simulink model "fuck"  (R2016a)
settings: Solver=ode5  StartTime=0.0  StopTime=10  FixedStep=0.001  RelTol=1e-3
values from neighbouring files (symbols this model uses):
  LK1 = -LK1    [car.m]    (also in car_m.m = [-1 0;0 -1]')
  x0 = [1 3 2 1 3 2 4 5]'    [car.m]    (also in car_m.m = [0 0]')
  xd = [10 10]    [car_m.m]
libraries: simulink x3
settings Model: Creator=108  LastModifiedBy=108

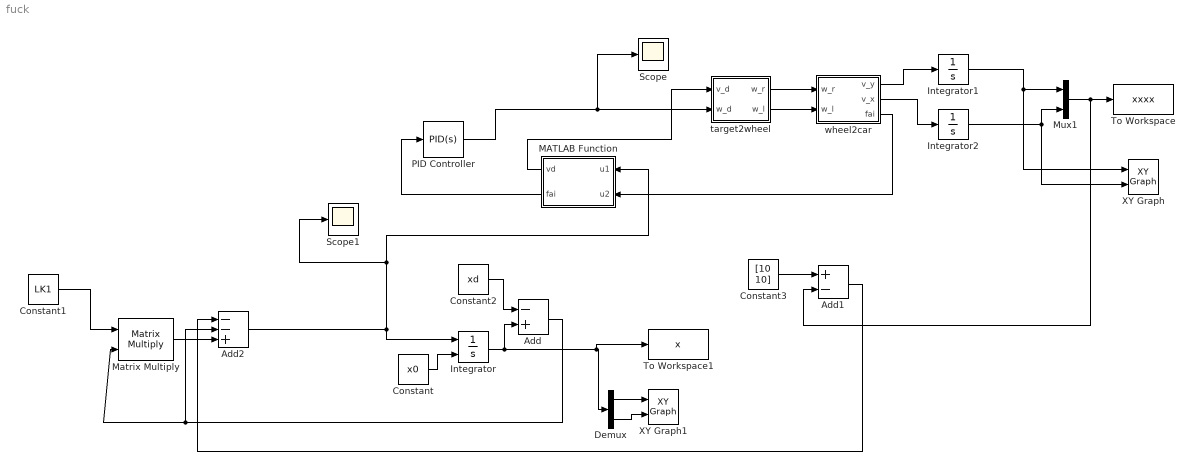
== system fuck ==
  Add : Sum  Inputs=-+
  Add1 : Sum  Inputs=+-
  Add2 : Sum  Inputs=--+
  Constant : Constant  Value=x0
  Constant1 : Constant  Value=LK1  VectorParams1D=off
  Constant2 : Constant  Value=xd
  Constant3 : Constant  Value=[10 10]
  Demux : Demux  Outputs=2
  Integrator : Integrator  InitialConditionSource=external
  Integrator1 : Integrator
  Integrator2 : Integrator
  MATLAB Function : MATLAB Function  TreatAsAtomicUnit=on
  Matrix Multiply : Product  Multiplication=Matrix(*)
  Mux1 : Mux  Inputs=2
  PID Controller : simulink/Continuous/PID Controller  Controller=PID  TimeDomain=Continuous-time  SampleTime=-1  IntegratorMethod=Forward Euler  FilterMethod=Forward Euler  Form=Parallel  UseFilter=on  ControllerParametersSource=internal  P=2  I=1  D=0  N=100  InitialConditionSource=internal  InitialConditionForIntegrator=0  InitialConditionForFilter=0  ExternalReset=none  LimitOutput=off  UpperSaturationLimit=inf  LowerSaturationLimit=-inf  LinearizeAsGain=on  AntiWindupMode=none  Kb=1  TrackingMode=off  Kt=1  PParamMin=[]  PParamMax=[]  IParamMin=[]  IParamMax=[]  DParamMin=[]  DParamMax=[]  NParamMin=[]  NParamMax=[]  KbParamMin=[]  KbParamMax=[]  KtParamMin=[]  KtParamMax=[]  POutMin=[]  POutMax=[]  IOutMin=[]  IOutMax=[]  DOutMin=[]  DOutMax=[]  NOutMin=[]  NOutMax=[]  KbOutMin=[]  KbOutMax=[]  KtOutMin=[]  KtOutMax=[]  IntegratorOutMin=[]  IntegratorOutMax=[]  FilterOutMin=[]  FilterOutMax=[]  SumOutMin=[]  SumOutMax=[]  SumI1OutMin=[]  SumI1OutMax=[]  SumI2OutMin=[]  SumI2OutMax=[]  SumI3OutMin=[]  SumI3OutMax=[]  SumDOutMin=[]  SumDOutMax=[]  SaturationOutMin=[]  SaturationOutMax=[]  IntegratorContinuousStateAttributes=''  IntegratorStateMustResolveToSignalObject=off  IntegratorRTWStateStorageClass=Auto  FilterContinuousStateAttributes=''  FilterStateMustResolveToSignalObject=off  FilterRTWStateStorageClass=Auto  DifferentiatorICPrevScaledInput=0  DifferentiatorOutMin=[]  DifferentiatorOutMax=[]
  Scope : Scope
  Scope1 : Scope
  To Workspace : ToWorkspace  VariableName=xxxx  SampleTime=-1
  To Workspace1 : ToWorkspace  VariableName=x  SampleTime=-1
  XY Graph : simulink/Sinks/XY Graph  xmin=-20  xmax=20  ymin=-20  ymax=20  st=0
  XY Graph1 : simulink/Sinks/XY Graph  xmin=-20  xmax=20  ymin=-20  ymax=20  st=0
  target2wheel : Subsystem
  wheel2car : Subsystem
  wires:
  Integrator1/1 -> Mux1/1, XY Graph/1
  Integrator2/1 -> Mux1/2, XY Graph/2
  wheel2car/1(v_y) -> Integrator1/1
  wheel2car/2(v_x) -> Integrator2/1
  target2wheel/1(w_r) -> wheel2car/1(w_r)
  target2wheel/2(w_l) -> wheel2car/2(w_l)
  Constant/1 -> Integrator/2
  Constant1/1 -> Matrix Multiply/1
  Integrator/1 -> Add/2, To Workspace1/1, Demux/1
  MATLAB Function/1(vd) -> target2wheel/1(v_d)
  Constant2/1 -> Add/1
  Add/1 -> Add2/2, Matrix Multiply/2
  MATLAB Function/2(fai) -> PID Controller/1
  PID Controller/1 -> Scope/1, target2wheel/2(w_d)
  wheel2car/3(fai) -> MATLAB Function/2(u2)
  Demux/1 -> XY Graph1/1
  Demux/2 -> XY Graph1/2
  Mux1/1 -> Add1/2, To Workspace/1
  Constant3/1 -> Add1/1
  Matrix Multiply/1 -> Add2/3
  Add2/1 -> Integrator/1, MATLAB Function/1(u1), Scope1/1
  Add1/1 -> Add2/1

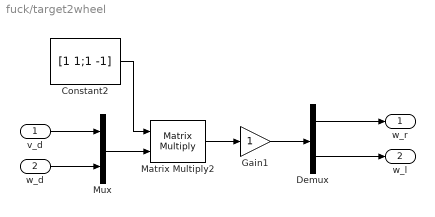
== system fuck/target2wheel ==
  v_d : Inport
  w_d : Inport  Port=2
  Constant2 : Constant  Value=[1 1;1 -1]
  Demux : Demux  Outputs=2
  Gain1 : Gain
  Matrix Multiply2 : Product  Multiplication=Matrix(*)
  Mux : Mux  Inputs=2
  w_r : Outport
  w_l : Outport  Port=2
  wires:
  Mux/1 -> Matrix Multiply2/2
  Gain1/1 -> Demux/1
  Constant2/1 -> Matrix Multiply2/1
  Matrix Multiply2/1 -> Gain1/1
  v_d/1 -> Mux/1
  w_d/1 -> Mux/2
  Demux/2 -> w_l/1
  Demux/1 -> w_r/1

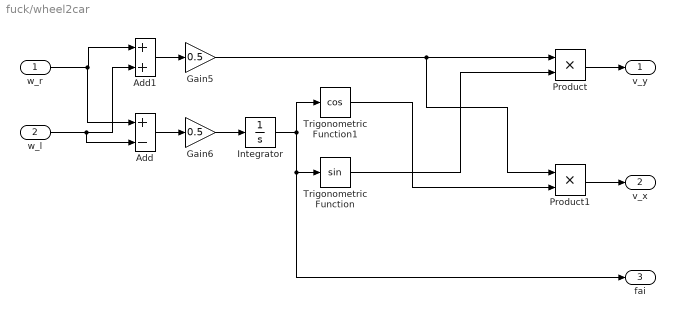
== system fuck/wheel2car ==
  w_r : Inport
  w_l : Inport  Port=2
  Add : Sum  Inputs=+-
  Add1 : Sum
  Gain5 : Gain  Gain=0.5
  Gain6 : Gain  Gain=0.5
  Integrator : Integrator
  Product : Product
  Product1 : Product
  Trigonometric Function : Trigonometry
  Trigonometric Function1 : Trigonometry  Operator=cos
  v_y : Outport
  v_x : Outport  Port=2
  fai : Outport  Port=3
  wires:
  Gain5/1 -> Product1/1, Product/1
  Gain6/1 -> Integrator/1
  Integrator/1 -> Trigonometric Function1/1, fai/1, Trigonometric Function/1
  Trigonometric Function/1 -> Product/2
  Trigonometric Function1/1 -> Product1/2
  Product/1 -> v_y/1
  w_r/1 -> Add/1, Add1/1
  w_l/1 -> Add/2, Add1/2
  Product1/1 -> v_x/1
  Add1/1 -> Gain5/1
  Add/1 -> Gain6/1

== matlab function fuck/MATLAB Function ==
  data: u1 input; vd output; fai output; u2 input
function [vd,fai]  = fcn(u1,u2)
%#codegen

vd=[0];
fai=[0];
fai_real=u2;
j=1;
for i=1:1
   vd(j) = sqrt(u1(i).^2+ u1(i+1).^2);
   fai_d = atan(u1(i+1)/u1(i));
   %fai_real(j) = atan(u2(i+1)/u2(i));
   j=j+1;
end
   fai= fai_d-fai_real;
end
